simulink model "SM_5_2016a"  (R2016a)
settings: Solver=ode15s  SolverMode=SingleTasking  StartTime=0.001  StopTime=10.0  FixedStep=0.0001  RelTol=1e-6
settings Model: Creator=guaca  LastModifiedBy=Guacamole
settings DebuggingCC: SFUnexpectedBacktrackingDiag=error  SFNoUnconditionalDefaultTransitionDiag=error
settings GRTTargetCC: TargetLangStandard=C99 (ISO)  GeneratePreprocessorConditionals=Use local settings
settings ConfigComp: CovMetricSettings=dwe  CovHtmlReporting=off  CovSaveCumulativeToWorkspaceVar=off  CovSaveSingleToWorkspaceVar=off  CovExternalEMLEnable=on

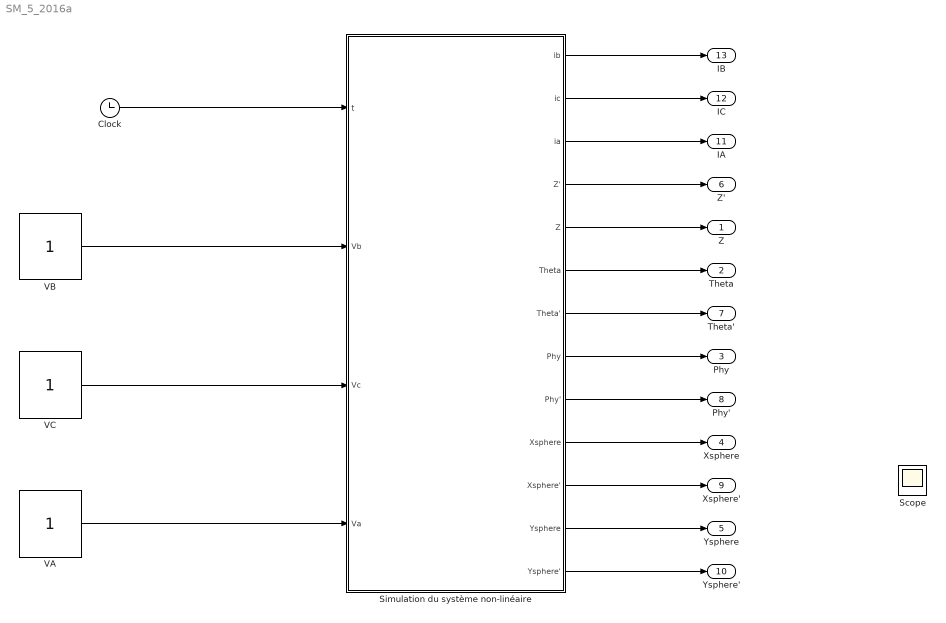
== system SM_5_2016a ==
  Clock : Clock
  Simulation du système non-linéaire : Subsystem
  VA : Constant
  VB : Constant
  VC : Constant
  Z : Outport
  Theta : Outport  Port=2
  Phy : Outport  Port=3
  Xsphere : Outport  Port=4
  Ysphere : Outport  Port=5
  Z' : Outport  Port=6
  Theta' : Outport  Port=7
  Phy' : Outport  Port=8
  Xsphere' : Outport  Port=9
  Ysphere' : Outport  Port=10
  IA : Outport  Port=11
  IC : Outport  Port=12
  IB : Outport  Port=13
  Scope : Scope
  wires:
  Clock/1 -> Simulation du système non-linéaire/1(t)
  VB/1 -> Simulation du système non-linéaire/2(Vb)
  VC/1 -> Simulation du système non-linéaire/3(Vc)
  VA/1 -> Simulation du système non-linéaire/4(Va)
  Simulation du système non-linéaire/1(ib) -> IB/1
  Simulation du système non-linéaire/2(ic) -> IC/1
  Simulation du système non-linéaire/3(ia) -> IA/1
  Simulation du système non-linéaire/4(Z') -> Z'/1
  Simulation du système non-linéaire/5(Z) -> Z/1
  Simulation du système non-linéaire/6(Theta) -> Theta/1
  Simulation du système non-linéaire/7(Theta') -> Theta'/1
  Simulation du système non-linéaire/8(Phy) -> Phy/1
  Simulation du système non-linéaire/9(Phy') -> Phy'/1
  Simulation du système non-linéaire/10(Xsphere) -> Xsphere/1
  Simulation du système non-linéaire/11(Xsphere') -> Xsphere'/1
  Simulation du système non-linéaire/12(Ysphere) -> Ysphere/1
  Simulation du système non-linéaire/13(Ysphere') -> Ysphere'/1

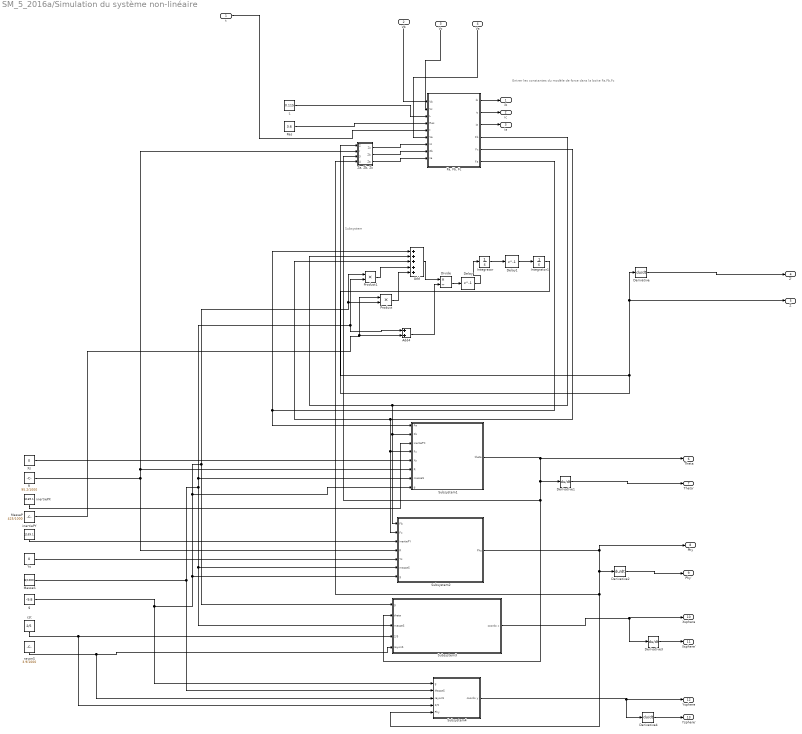
== system SM_5_2016a/Simulation du système non-linéaire ==
  note: Subsystem
  note: Entrer les constantes du modèle de force dans la boite Fa,Fb,Fc
  t : Inport
  Vb : Inport  Port=2
  Vc : Inport  Port=3
  Va : Inport  Port=4
  Add : Sum  Inputs=+++++
  Add4 : Sum
  Delay : Delay  DelayLength=1  InitialCondition=0
  Delay1 : Delay  DelayLength=1  InitialCondition=0
  Derivative{,1..4} (5 alike) : Derivative
  Divide : Product  Inputs=*/
  "Fa, Fb, Fc" : Subsystem
  Integrator : Integrator
  Integrator1 : Integrator
  L : Constant  Value=0.115
  MasseP : Constant  Value=425/1000
  MasseS : Constant  Value=8/1000
  Product : Product
  Product1 : Product
  R : Constant  Value=95.2/1000
  Res : Constant  Value=3.6
  Subsystem1 : Subsystem
  Subsystem2 : Subsystem
  Subsystem3 : Subsystem
  Subsystem4 : Subsystem
  Xs : Constant  Value=0
  Ys : Constant  Value=0
  "Za, Zb, Zc" : Subsystem
  cst : Constant  Value=2/5
  g : Constant  Value=-9.8
  inertiePX : Constant  Value=1169.1
  inertiePY : Constant  Value=1169.1
  rayonS : Constant  Value=3.9/1000
  ib : Outport
  ic : Outport  Port=2
  ia : Outport  Port=3
  Z' : Outport  Port=4
  Z : Outport  Port=5
  Theta : Outport  Port=6
  Theta' : Outport  Port=7
  Phy : Outport  Port=8
  Phy' : Outport  Port=9
  Xsphere : Outport  Port=10
  Xsphere' : Outport  Port=11
  Ysphere : Outport  Port=12
  Ysphere' : Outport  Port=13
  wires:
  rayonS/1 -> Subsystem3/5(rayonS), Subsystem4/3(rayonS)
  R/1 -> Subsystem2/4(R), "Za, Zb, Zc"/2(r), Subsystem1/6(R)
  cst/1 -> Subsystem4/4(2/5), Subsystem3/4(2/5)
  Subsystem1/1(theta) -> Theta/1, "Za, Zb, Zc"/3(Theta), Subsystem3/2(theta), Derivative1/1
  inertiePX/1 -> Subsystem1/3(inertiePX)
  Ys/1 -> Subsystem2/5(Ys)
  Xs/1 -> Subsystem1/5(Xs)
  Subsystem2/1(Phy) -> Phy/1, "Za, Zb, Zc"/4(phy), Subsystem4/5(Phy), Derivative2/1
  Subsystem3/1(coordo x) -> Xsphere/1, Derivative3/1
  Subsystem4/1(coordo y) -> Ysphere/1, Derivative4/1
  inertiePY/1 -> Subsystem2/3(inertiePY)
  Derivative2/1 -> Phy'/1
  t/1 -> "Fa, Fb, Fc"/5(t)
  Va/1 -> "Fa, Fb, Fc"/6(Va)
  Res/1 -> "Fa, Fb, Fc"/4(Res)
  "Fa, Fb, Fc"/2(ic) -> ic/1
  "Fa, Fb, Fc"/3(ia) -> ia/1
  Derivative1/1 -> Theta'/1
  "Fa, Fb, Fc"/1(ib) -> ib/1
  L/1 -> "Fa, Fb, Fc"/3(L)
  Vc/1 -> "Fa, Fb, Fc"/2(Vc)
  Vb/1 -> "Fa, Fb, Fc"/1(Vb)
  Derivative/1 -> Z'/1
  "Za, Zb, Zc"/1(Zc) -> "Fa, Fb, Fc"/7(zc)
  "Za, Zb, Zc"/2(Zb) -> "Fa, Fb, Fc"/8(Zb)
  "Za, Zb, Zc"/3(Za) -> "Fa, Fb, Fc"/9(za)
  Derivative3/1 -> Xsphere'/1
  Integrator1/1 -> Derivative/1, Z/1, "Za, Zb, Zc"/1(Z)
  Derivative4/1 -> Ysphere'/1
  Delay1/1 -> Integrator1/1
  Delay/1 -> Integrator/1
  MasseS/1 -> Subsystem4/2(MasseS), Subsystem3/3(masseS), Subsystem2/6(masseS), Product1/2, Add4/1, Subsystem1/7(masseS)
  g/1 -> Product1/1, Product/2, Subsystem3/1(g), Subsystem1/8(g), Subsystem2/7(g), Subsystem4/1(g)
  "Fa, Fb, Fc"/5(Fc) -> Add/3, Subsystem2/2(Fc), Subsystem1/4(Fc)
  "Fa, Fb, Fc"/4(Fb) -> Add/2, Subsystem2/1(Fb), Subsystem1/2(Fb)
  "Fa, Fb, Fc"/6(Fa) -> Add/1, Subsystem1/1(Fa)
  Add4/1 -> Divide/2
  Add/1 -> Divide/1
  Product1/1 -> Add/4
  Product/1 -> Add/5
  MasseP/1 -> Add4/2, Product/1
  Integrator/1 -> Delay1/1
  Divide/1 -> Delay/1

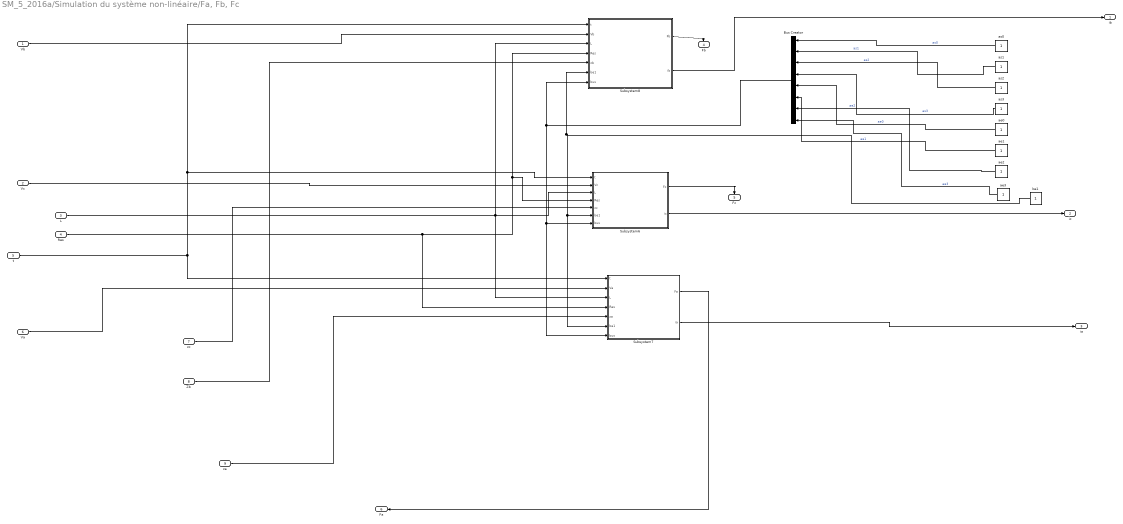
== system SM_5_2016a/Simulation du système non-linéaire/Fa, Fb, Fc ==
  Vb : Inport
  Vc : Inport  Port=2
  L : Inport  Port=3
  Res : Inport  Port=4
  t : Inport  Port=5
  Va : Inport  Port=6
  zc : Inport  Port=7
  Zb : Inport  Port=8
  za : Inport  Port=9
  Bus Creator : BusCreator  Inputs='as0','as1','as2','as3','ae0','ae1','ae2','ae3'
  Subsystem6 : Subsystem
  Subsystem7 : Subsystem
  Subsystem8 : Subsystem
  ae{0..3} (4 alike) : Constant
  as{0..3} (4 alike) : Constant
  be1 : Constant
  ib : Outport
  ic : Outport  Port=2
  ia : Outport  Port=3
  Fb : Outport  Port=4
  Fc : Outport  Port=5
  Fa : Outport  Port=6
  wires:
  ae1/1 -> Bus Creator/6  "ae1"
  ae0/1 -> Bus Creator/5  "ae0"
  as2/1 -> Bus Creator/3  "as2"
  as3/1 -> Bus Creator/4  "as3"
  za/1 -> Subsystem7/5(za)
  Bus Creator/1 -> Subsystem7/7(bus), Subsystem6/7(bus), Subsystem8/7(bus)
  Va/1 -> Subsystem7/2(Va)
  Zb/1 -> Subsystem8/5(zb)
  zc/1 -> Subsystem6/5(zc)
  Subsystem6/1(Fc) -> Fc/1
  be1/1 -> Subsystem7/6(be1), Subsystem6/6(be1), Subsystem8/6(be1)
  Subsystem8/1(Fb) -> Fb/1
  Vb/1 -> Subsystem8/2(Vb)
  Vc/1 -> Subsystem6/2(Vc)
  L/1 -> Subsystem7/3(L), Subsystem6/3(L), Subsystem8/3(L)
  Res/1 -> Subsystem7/4(Res), Subsystem6/4(Res), Subsystem8/4(Res)
  t/1 -> Subsystem8/1(t), Subsystem6/1(t), Subsystem7/1(t)
  as0/1 -> Bus Creator/1  "as0"
  Subsystem7/1(Fa) -> Fa/1
  ae2/1 -> Bus Creator/7  "ae2"
  ae3/1 -> Bus Creator/8  "ae3"
  as1/1 -> Bus Creator/2  "as1"
  Subsystem7/2(ia) -> ia/1
  Subsystem8/2(ib) -> ib/1
  Subsystem6/2(ic) -> ic/1

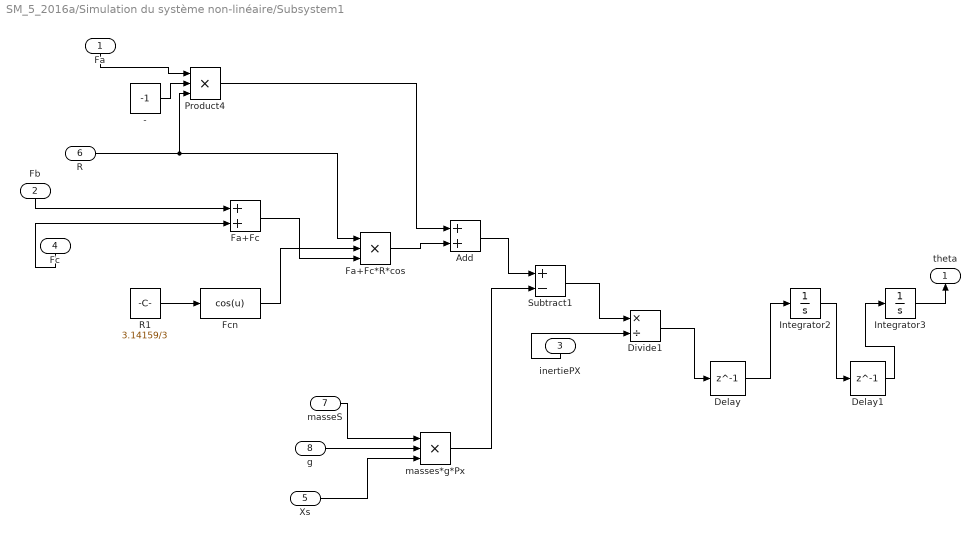
== system SM_5_2016a/Simulation du système non-linéaire/Subsystem1 ==
  Fa : Inport
  Fb : Inport  Port=2
  inertiePX : Inport  Port=3
  Fc : Inport  Port=4
  Xs : Inport  Port=5
  R : Inport  Port=6
  masseS : Inport  Port=7
  g : Inport  Port=8
  - : Constant  Value=-1
  Add : Sum
  Delay : Delay  DelayLength=1  InitialCondition=0
  Delay1 : Delay  DelayLength=1  InitialCondition=0
  Divide1 : Product  Inputs=*/
  Fa+Fc : Sum
  Fa+Fc*R*cos : Product  Inputs=3
  Fcn : Fcn  Expr=cos(u)
  Integrator2 : Integrator
  Integrator3 : Integrator
  Product4 : Product  Inputs=3
  R1 : Constant  Value=3.14159/3
  Subtract1 : Sum  Inputs=+-
  masses*g*Px : Product  Inputs=3
  theta : Outport
  wires:
  Fa+Fc/1 -> Fa+Fc*R*cos/3
  Product4/1 -> Add/1
  -/1 -> Product4/2
  Add/1 -> Subtract1/1
  Subtract1/1 -> Divide1/1
  inertiePX/1 -> Divide1/2
  Divide1/1 -> Delay/1
  Integrator2/1 -> Delay1/1
  Integrator3/1 -> theta/1
  R1/1 -> Fcn/1
  R/1 -> Fa+Fc*R*cos/1, Product4/3
  Fcn/1 -> Fa+Fc*R*cos/2
  Fa+Fc*R*cos/1 -> Add/2
  Xs/1 -> masses*g*Px/3
  masses*g*Px/1 -> Subtract1/2
  masseS/1 -> masses*g*Px/1
  g/1 -> masses*g*Px/2
  Fc/1 -> Fa+Fc/2
  Fb/1 -> Fa+Fc/1
  Fa/1 -> Product4/1
  Delay/1 -> Integrator2/1
  Delay1/1 -> Integrator3/1

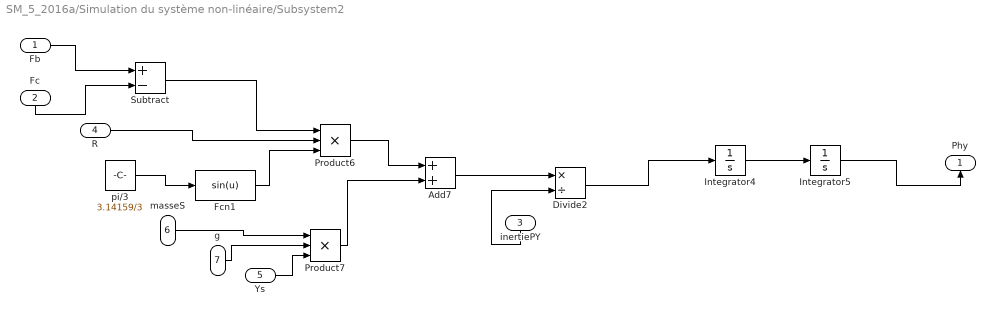
== system SM_5_2016a/Simulation du système non-linéaire/Subsystem2 ==
  Fb : Inport
  Fc : Inport  Port=2
  inertiePY : Inport  Port=3
  R : Inport  Port=4
  Ys : Inport  Port=5
  masseS : Inport  Port=6
  g : Inport  Port=7
  Add7 : Sum
  Divide2 : Product  Inputs=*/
  Fcn1 : Fcn  Expr=sin(u)
  Integrator4 : Integrator
  Integrator5 : Integrator
  Product6 : Product  Inputs=3
  Product7 : Product  Inputs=3
  Subtract : Sum  Inputs=+-
  pi/3 : Constant  Value=3.14159/3
  Phy : Outport
  wires:
  Fcn1/1 -> Product6/3
  pi/3/1 -> Fcn1/1
  Subtract/1 -> Product6/1
  Product6/1 -> Add7/1
  Product7/1 -> Add7/2
  Add7/1 -> Divide2/1
  inertiePY/1 -> Divide2/2
  Divide2/1 -> Integrator4/1
  Integrator4/1 -> Integrator5/1
  Integrator5/1 -> Phy/1
  masseS/1 -> Product7/1
  Fc/1 -> Subtract/2
  Ys/1 -> Product7/3
  R/1 -> Product6/2
  g/1 -> Product7/2
  Fb/1 -> Subtract/1

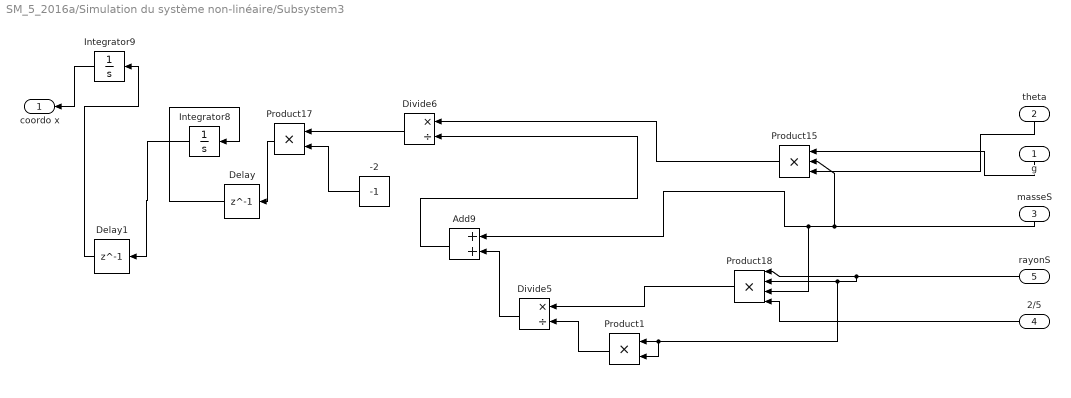
== system SM_5_2016a/Simulation du système non-linéaire/Subsystem3 ==
  g : Inport
  theta : Inport  Port=2
  masseS : Inport  Port=3
  2/5 : Inport  Port=4
  rayonS : Inport  Port=5
  -2 : Constant  Value=-1
  Add9 : Sum
  Delay : Delay  DelayLength=1  InitialCondition=0
  Delay1 : Delay  DelayLength=1  InitialCondition=0
  Divide5 : Product  Inputs=*/
  Divide6 : Product  Inputs=*/
  Integrator8 : Integrator
  Integrator9 : Integrator
  Product1 : Product
  Product15 : Product  Inputs=3
  Product17 : Product
  Product18 : Product  Inputs=4
  coordo x : Outport
  wires:
  Product18/1 -> Divide5/1
  Divide5/1 -> Add9/2
  Product15/1 -> Divide6/1
  Add9/1 -> Divide6/2
  Integrator8/1 -> Delay1/1
  Integrator9/1 -> coordo x/1
  Divide6/1 -> Product17/1
  -2/1 -> Product17/2
  masseS/1 -> Product15/2, Add9/1, Product18/3
  rayonS/1 -> Product1/2, Product1/1, Product18/2, Product18/1
  2/5/1 -> Product18/4
  g/1 -> Product15/1
  theta/1 -> Product15/3
  Product17/1 -> Delay/1
  Delay/1 -> Integrator8/1
  Delay1/1 -> Integrator9/1
  Product1/1 -> Divide5/2

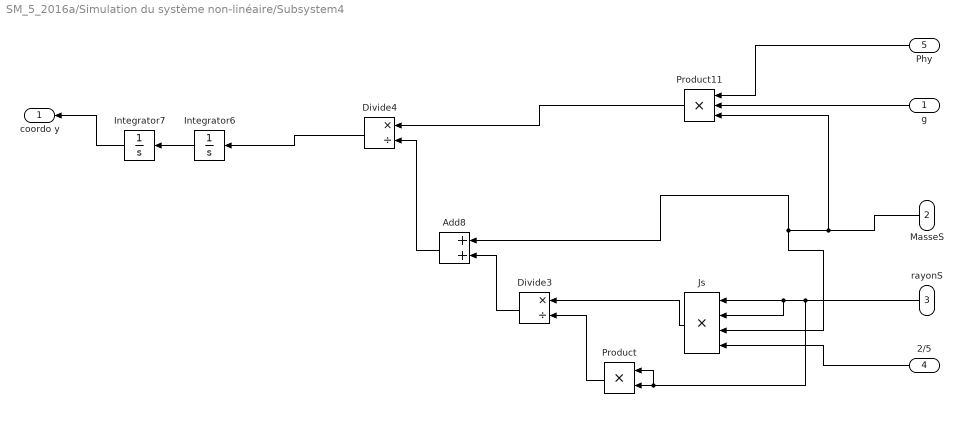
== system SM_5_2016a/Simulation du système non-linéaire/Subsystem4 ==
  g : Inport
  MasseS : Inport  Port=2
  rayonS : Inport  Port=3
  2/5 : Inport  Port=4
  Phy : Inport  Port=5
  Add8 : Sum
  Divide3 : Product  Inputs=*/
  Divide4 : Product  Inputs=*/
  Integrator6 : Integrator
  Integrator7 : Integrator
  Js : Product  Inputs=4
  Product : Product
  Product11 : Product  Inputs=3
  coordo y : Outport
  wires:
  Js/1 -> Divide3/1
  Divide3/1 -> Add8/2
  Product11/1 -> Divide4/1
  Add8/1 -> Divide4/2
  Integrator6/1 -> Integrator7/1
  Integrator7/1 -> coordo y/1
  Divide4/1 -> Integrator6/1
  g/1 -> Product11/2
  rayonS/1 -> Product/1, Product/2, Js/2, Js/1
  2/5/1 -> Js/4
  Phy/1 -> Product11/1
  MasseS/1 -> Product11/3, Js/3, Add8/1
  Product/1 -> Divide3/2

== system SM_5_2016a/Simulation du système non-linéaire/Za, Zb, Zc ==
  Z : Inport
  r : Inport  Port=2
  Theta : Inport  Port=3
  phy : Inport  Port=4
  Subsystem10 : Subsystem
  Subsystem5 : Subsystem
  Subsystem9 : Subsystem
  Zc : Outport
  Zb : Outport  Port=2
  Za : Outport  Port=3
  wires:
  Subsystem5/1(Za) -> Za/1
  Subsystem10/1(Zc) -> Zc/1
  Subsystem9/1(Zb) -> Zb/1
  r/1 -> Subsystem10/3(r), Subsystem9/3(r), Subsystem5/3(R)
  phy/1 -> Subsystem10/4(phy), Subsystem9/4(phy)
  Z/1 -> Subsystem10/1(Z), Subsystem9/1(Z), Subsystem5/1(Z)
  Theta/1 -> Subsystem10/2(theta), Subsystem9/2(theta), Subsystem5/2(theta)

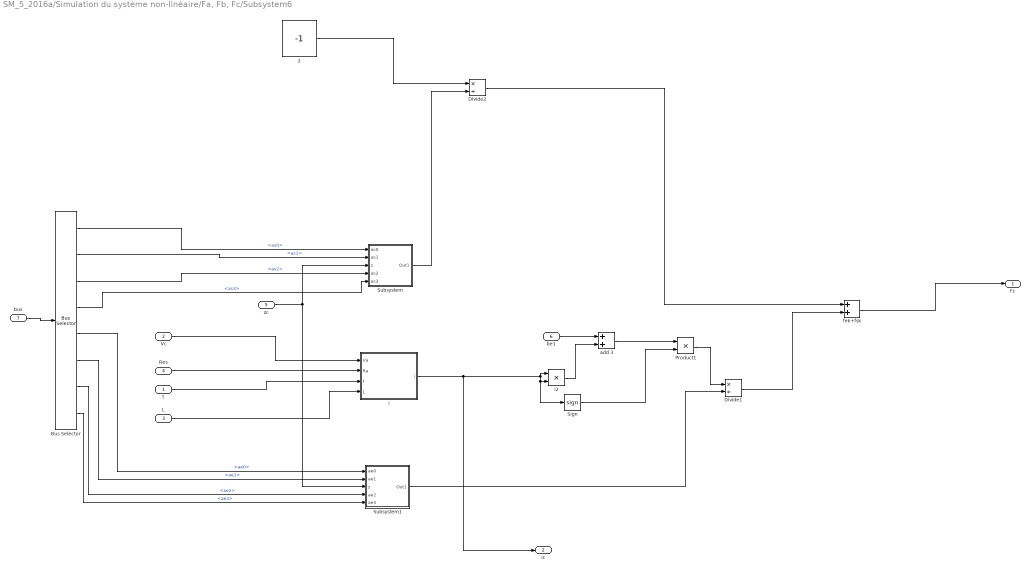
== system SM_5_2016a/Simulation du système non-linéaire/Fa, Fb, Fc/Subsystem6 ==
  t : Inport
  Vc : Inport  Port=2
  L : Inport  Port=3
  Res : Inport  Port=4
  zc : Inport  Port=5
  be1 : Inport  Port=6
  bus : Inport  Port=7
  2 : Constant  Value=-1
  Bus Selector : BusSelector  OutputSignals=as0,as1,as2,as3,ae0,ae1,ae2,ae3
  Divide1 : Product  Inputs=*/
  Divide2 : Product  Inputs=*/
  Product1 : Product
  Sign : Signum
  Subsystem : Subsystem
  Subsystem1 : Subsystem
  add 3 : Sum
  fek+fsk : Sum
  i : Subsystem
  i2 : Product
  Fc : Outport
  ic : Outport  Port=2
  wires:
  fek+fsk/1 -> Fc/1
  2/1 -> Divide2/1
  Divide2/1 -> fek+fsk/1
  i2/1 -> add 3/2
  i/1(i) -> ic/1, Sign/1, i2/2, i2/1
  Vc/1 -> i/1(Va)
  Res/1 -> i/2(Ra)
  t/1 -> i/3(t)
  L/1 -> i/4(L)
  be1/1 -> add 3/1
  add 3/1 -> Product1/1
  Sign/1 -> Product1/2
  Bus Selector/1 -> Subsystem/1(as0)  "<as0>"
  Bus Selector/2 -> Subsystem/2(as1)  "<as1>"
  zc/1 -> Subsystem/3(z), Subsystem1/3(z)
  Bus Selector/3 -> Subsystem/4(as2)  "<as2>"
  Bus Selector/4 -> Subsystem/5(as3)  "<as3>"
  Subsystem/1(Out1) -> Divide2/2
  Bus Selector/5 -> Subsystem1/1(ae0)  "<ae0>"
  Bus Selector/6 -> Subsystem1/2(ae1)  "<ae1>"
  Bus Selector/7 -> Subsystem1/4(ae2)  "<ae2>"
  Bus Selector/8 -> Subsystem1/5(ae3)  "<ae3>"
  Subsystem1/1(Out1) -> Divide1/2
  Product1/1 -> Divide1/1
  Divide1/1 -> fek+fsk/2
  bus/1 -> Bus Selector/1

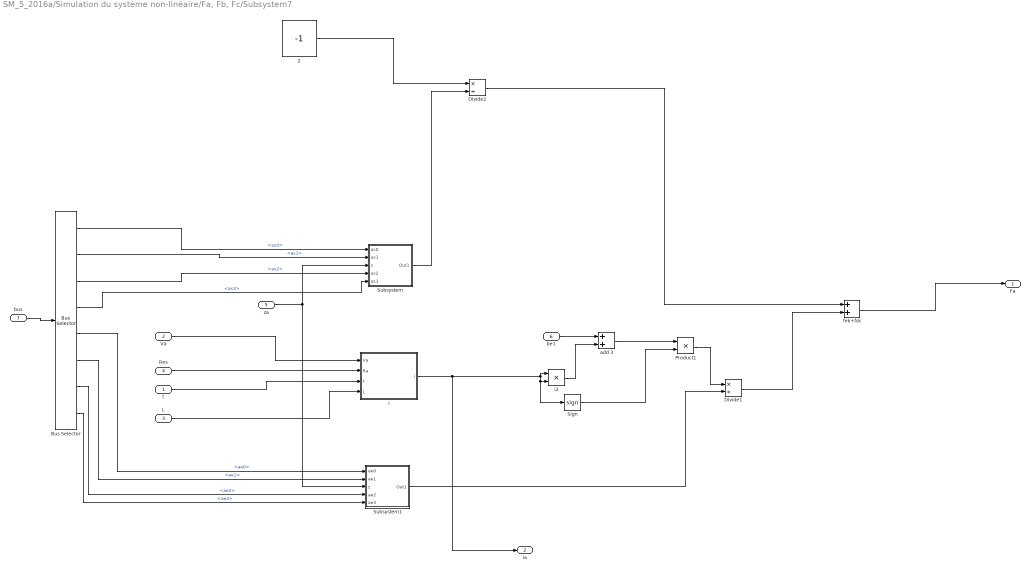
== system SM_5_2016a/Simulation du système non-linéaire/Fa, Fb, Fc/Subsystem7 ==
  t : Inport
  Va : Inport  Port=2
  L : Inport  Port=3
  Res : Inport  Port=4
  za : Inport  Port=5
  be1 : Inport  Port=6
  bus : Inport  Port=7
  2 : Constant  Value=-1
  Bus Selector : BusSelector  OutputSignals=as0,as1,as2,as3,ae0,ae1,ae2,ae3
  Divide1 : Product  Inputs=*/
  Divide2 : Product  Inputs=*/
  Product1 : Product
  Sign : Signum
  Subsystem : Subsystem
  Subsystem1 : Subsystem
  add 3 : Sum
  fek+fsk : Sum
  i : Subsystem
  i2 : Product
  Fa : Outport
  ia : Outport  Port=2
  wires:
  fek+fsk/1 -> Fa/1
  2/1 -> Divide2/1
  Divide2/1 -> fek+fsk/1
  i2/1 -> add 3/2
  i/1(i) -> ia/1, Sign/1, i2/2, i2/1
  Va/1 -> i/1(Va)
  Res/1 -> i/2(Ra)
  t/1 -> i/3(t)
  L/1 -> i/4(L)
  be1/1 -> add 3/1
  add 3/1 -> Product1/1
  Sign/1 -> Product1/2
  Bus Selector/1 -> Subsystem/1(as0)  "<as0>"
  Bus Selector/2 -> Subsystem/2(as1)  "<as1>"
  za/1 -> Subsystem/3(z), Subsystem1/3(z)
  Bus Selector/3 -> Subsystem/4(as2)  "<as2>"
  Bus Selector/4 -> Subsystem/5(as3)  "<as3>"
  Subsystem/1(Out1) -> Divide2/2
  Bus Selector/5 -> Subsystem1/1(ae0)  "<ae0>"
  Bus Selector/6 -> Subsystem1/2(ae1)  "<ae1>"
  Bus Selector/7 -> Subsystem1/4(ae2)  "<ae2>"
  Bus Selector/8 -> Subsystem1/5(ae3)  "<ae3>"
  Subsystem1/1(Out1) -> Divide1/2
  Product1/1 -> Divide1/1
  Divide1/1 -> fek+fsk/2
  bus/1 -> Bus Selector/1

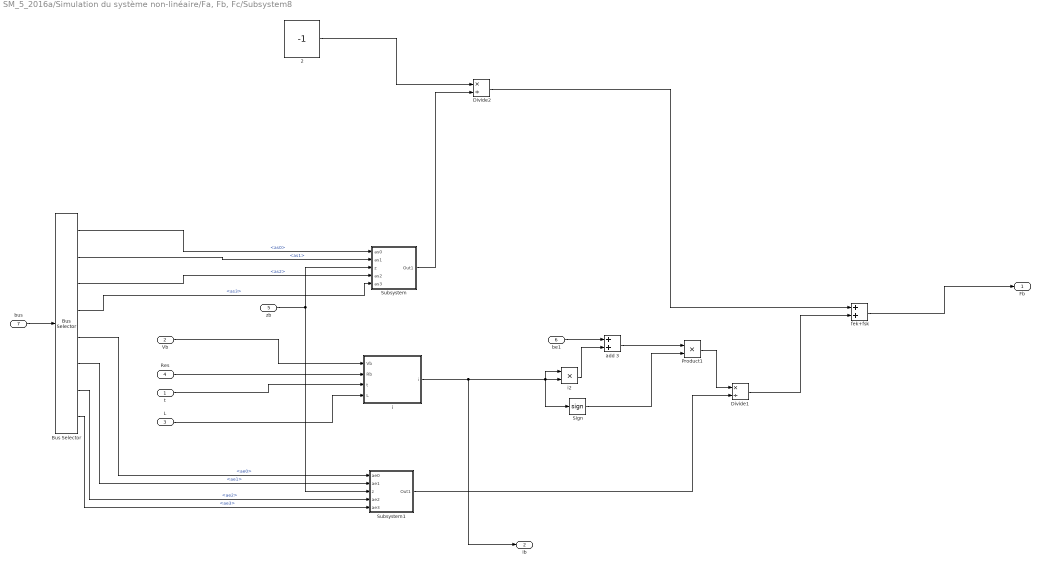
== system SM_5_2016a/Simulation du système non-linéaire/Fa, Fb, Fc/Subsystem8 ==
  t : Inport
  Vb : Inport  Port=2
  L : Inport  Port=3
  Res : Inport  Port=4
  zb : Inport  Port=5
  be1 : Inport  Port=6
  bus : Inport  Port=7
  2 : Constant  Value=-1
  Bus Selector : BusSelector  OutputSignals=as0,as1,as2,as3,ae0,ae1,ae2,ae3
  Divide1 : Product  Inputs=*/
  Divide2 : Product  Inputs=*/
  Product1 : Product
  Sign : Signum
  Subsystem : Subsystem
  Subsystem1 : Subsystem
  add 3 : Sum
  fek+fsk : Sum
  i : Subsystem
  i2 : Product
  Fb : Outport
  ib : Outport  Port=2
  wires:
  fek+fsk/1 -> Fb/1
  2/1 -> Divide2/1
  Divide2/1 -> fek+fsk/1
  i2/1 -> add 3/2
  i/1(i) -> ib/1, Sign/1, i2/2, i2/1
  Vb/1 -> i/1(Vb)
  Res/1 -> i/2(Rb)
  t/1 -> i/3(t)
  L/1 -> i/4(L)
  be1/1 -> add 3/1
  add 3/1 -> Product1/1
  Sign/1 -> Product1/2
  Bus Selector/1 -> Subsystem/1(as0)  "<as0>"
  Bus Selector/2 -> Subsystem/2(as1)  "<as1>"
  zb/1 -> Subsystem/3(z), Subsystem1/3(z)
  Bus Selector/3 -> Subsystem/4(as2)  "<as2>"
  Bus Selector/4 -> Subsystem/5(as3)  "<as3>"
  Subsystem/1(Out1) -> Divide2/2
  Bus Selector/5 -> Subsystem1/1(ae0)  "<ae0>"
  Bus Selector/6 -> Subsystem1/2(ae1)  "<ae1>"
  Bus Selector/7 -> Subsystem1/4(ae2)  "<ae2>"
  Bus Selector/8 -> Subsystem1/5(ae3)  "<ae3>"
  Subsystem1/1(Out1) -> Divide1/2
  Product1/1 -> Divide1/1
  Divide1/1 -> fek+fsk/2
  bus/1 -> Bus Selector/1

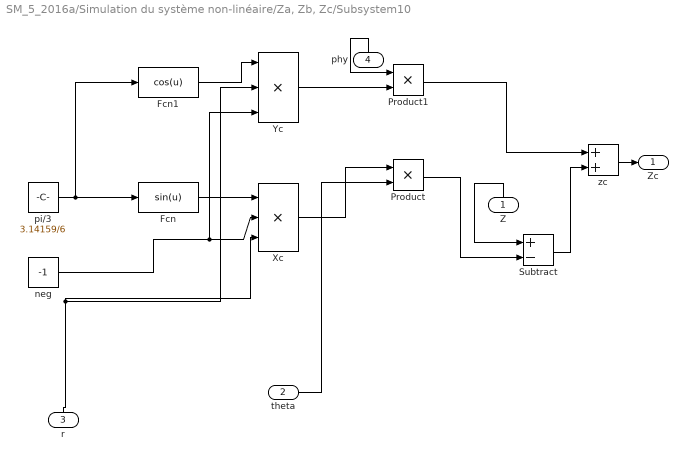
== system SM_5_2016a/Simulation du système non-linéaire/Za, Zb, Zc/Subsystem10 ==
  Z : Inport
  theta : Inport  Port=2
  r : Inport  Port=3
  phy : Inport  Port=4
  Fcn : Fcn  Expr=sin(u)
  Fcn1 : Fcn  Expr=cos(u)
  Product : Product
  Product1 : Product
  Subtract : Sum  Inputs=+-
  Xc : Product  Inputs=3
  Yc : Product  Inputs=3
  neg : Constant  Value=-1
  pi/3 : Constant  Value=3.14159/6
  zc : Sum
  Zc : Outport
  wires:
  Fcn1/1 -> Yc/1
  Xc/1 -> Product/1
  neg/1 -> Yc/3, Xc/2
  phy/1 -> Product1/1
  r/1 -> Yc/2, Xc/3
  zc/1 -> Zc/1
  Product1/1 -> zc/1
  Z/1 -> Subtract/1
  theta/1 -> Product/2
  Fcn/1 -> Xc/1
  pi/3/1 -> Fcn1/1, Fcn/1
  Product/1 -> Subtract/2
  Subtract/1 -> zc/2
  Yc/1 -> Product1/2

== system SM_5_2016a/Simulation du système non-linéaire/Za, Zb, Zc/Subsystem5 ==
  Z : Inport
  theta : Inport  Port=2
  R : Inport  Port=3
  Product : Product
  Subtract : Sum  Inputs=+-
  Za : Outport
  wires:
  Product/1 -> Subtract/2
  Subtract/1 -> Za/1
  Z/1 -> Subtract/1
  R/1 -> Product/1
  theta/1 -> Product/2

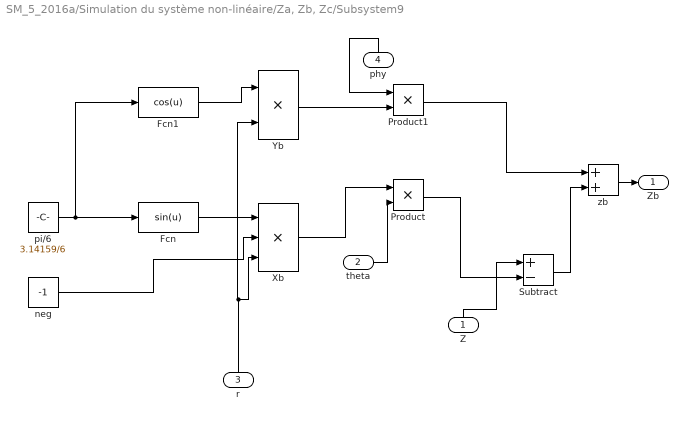
== system SM_5_2016a/Simulation du système non-linéaire/Za, Zb, Zc/Subsystem9 ==
  Z : Inport
  theta : Inport  Port=2
  r : Inport  Port=3
  phy : Inport  Port=4
  Fcn : Fcn  Expr=sin(u)
  Fcn1 : Fcn  Expr=cos(u)
  Product : Product
  Product1 : Product
  Subtract : Sum  Inputs=+-
  Xb : Product  Inputs=3
  Yb : Product
  neg : Constant  Value=-1
  pi/6 : Constant  Value=3.14159/6
  zb : Sum
  Zb : Outport
  wires:
  Fcn1/1 -> Yb/1
  Xb/1 -> Product/1
  neg/1 -> Xb/2
  phy/1 -> Product1/1
  r/1 -> Yb/2, Xb/3
  zb/1 -> Zb/1
  Product1/1 -> zb/1
  Z/1 -> Subtract/1
  theta/1 -> Product/2
  Fcn/1 -> Xb/1
  pi/6/1 -> Fcn1/1, Fcn/1
  Product/1 -> Subtract/2
  Subtract/1 -> zb/2
  Yb/1 -> Product1/2

== system SM_5_2016a/Simulation du système non-linéaire/Fa, Fb, Fc/Subsystem6/Subsystem ==
  as0 : Inport
  as1 : Inport  Port=2
  z : Inport  Port=3
  as2 : Inport  Port=4
  as3 : Inport  Port=5
  Add : Sum  Inputs=++++
  Product4 : Product
  Product5 : Product  Inputs=3
  Product6 : Product  Inputs=4
  Out1 : Outport
  wires:
  as0/1 -> Add/1
  Product5/1 -> Add/3
  Product4/1 -> Add/2
  Product6/1 -> Add/4
  z/1 -> Product5/3, Product6/1, Product6/4, Product6/3, Product5/1, Product4/1
  as1/1 -> Product4/2
  as2/1 -> Product5/2
  as3/1 -> Product6/2
  Add/1 -> Out1/1

== system SM_5_2016a/Simulation du système non-linéaire/Fa, Fb, Fc/Subsystem6/Subsystem1 ==
  ae0 : Inport
  ae1 : Inport  Port=2
  z : Inport  Port=3
  ae2 : Inport  Port=4
  ae3 : Inport  Port=5
  Add : Sum  Inputs=++++
  Product4 : Product
  Product5 : Product  Inputs=3
  Product6 : Product  Inputs=4
  Out1 : Outport
  wires:
  ae0/1 -> Add/1
  Product5/1 -> Add/3
  Product4/1 -> Add/2
  Product6/1 -> Add/4
  z/1 -> Product5/3, Product6/1, Product6/4, Product6/3, Product5/1, Product4/1
  ae1/1 -> Product4/2
  ae2/1 -> Product5/2
  ae3/1 -> Product6/2
  Add/1 -> Out1/1

== system SM_5_2016a/Simulation du système non-linéaire/Fa, Fb, Fc/Subsystem6/i ==
  Va : Inport
  Ra : Inport  Port=2
  t : Inport  Port=3
  L : Inport  Port=4
  1 : Constant
  3 : Constant  Value=-1
  Divide1 : Product  Inputs=*/
  Divide8 : Product  Inputs=*/
  Math Function : Math  SaturateOnIntegerOverflow=on
  Product1 : Product
  Product20 : Product
  Product3 : Product
  Subtract2 : Sum  Inputs=+-
  i : Outport
  wires:
  1/1 -> Subtract2/1
  Math Function/1 -> Subtract2/2
  Divide8/1 -> Math Function/1
  Va/1 -> Divide1/1
  Ra/1 -> Product20/1, Divide1/2
  t/1 -> Product20/2
  Product20/1 -> Divide8/1
  L/1 -> Product1/1
  3/1 -> Product1/2
  Product1/1 -> Divide8/2
  Divide1/1 -> Product3/1
  Subtract2/1 -> Product3/2
  Product3/1 -> i/1  "i"

== system SM_5_2016a/Simulation du système non-linéaire/Fa, Fb, Fc/Subsystem7/Subsystem ==
  as0 : Inport
  as1 : Inport  Port=2
  z : Inport  Port=3
  as2 : Inport  Port=4
  as3 : Inport  Port=5
  Add : Sum  Inputs=++++
  Product4 : Product
  Product5 : Product  Inputs=3
  Product6 : Product  Inputs=4
  Out1 : Outport
  wires:
  as0/1 -> Add/1
  Product5/1 -> Add/3
  Product4/1 -> Add/2
  Product6/1 -> Add/4
  z/1 -> Product5/3, Product6/1, Product6/4, Product6/3, Product5/1, Product4/1
  as1/1 -> Product4/2
  as2/1 -> Product5/2
  as3/1 -> Product6/2
  Add/1 -> Out1/1

== system SM_5_2016a/Simulation du système non-linéaire/Fa, Fb, Fc/Subsystem7/Subsystem1 ==
  ae0 : Inport
  ae1 : Inport  Port=2
  z : Inport  Port=3
  ae2 : Inport  Port=4
  ae3 : Inport  Port=5
  Add : Sum  Inputs=++++
  Product4 : Product
  Product5 : Product  Inputs=3
  Product6 : Product  Inputs=4
  Out1 : Outport
  wires:
  ae0/1 -> Add/1
  Product5/1 -> Add/3
  Product4/1 -> Add/2
  Product6/1 -> Add/4
  z/1 -> Product5/3, Product6/1, Product6/4, Product6/3, Product5/1, Product4/1
  ae1/1 -> Product4/2
  ae2/1 -> Product5/2
  ae3/1 -> Product6/2
  Add/1 -> Out1/1

== system SM_5_2016a/Simulation du système non-linéaire/Fa, Fb, Fc/Subsystem7/i ==
  Va : Inport
  Ra : Inport  Port=2
  t : Inport  Port=3
  L : Inport  Port=4
  1 : Constant
  3 : Constant  Value=-1
  Divide1 : Product  Inputs=*/
  Divide8 : Product  Inputs=*/
  Math Function : Math  SaturateOnIntegerOverflow=on
  Product1 : Product
  Product20 : Product
  Product3 : Product
  Subtract2 : Sum  Inputs=+-
  i : Outport
  wires:
  1/1 -> Subtract2/1
  Math Function/1 -> Subtract2/2
  Divide8/1 -> Math Function/1
  Va/1 -> Divide1/1
  Ra/1 -> Product20/1, Divide1/2
  t/1 -> Product20/2
  Product20/1 -> Divide8/1
  L/1 -> Product1/1
  3/1 -> Product1/2
  Product1/1 -> Divide8/2
  Divide1/1 -> Product3/1
  Subtract2/1 -> Product3/2
  Product3/1 -> i/1  "i"

== system SM_5_2016a/Simulation du système non-linéaire/Fa, Fb, Fc/Subsystem8/Subsystem ==
  as0 : Inport
  as1 : Inport  Port=2
  z : Inport  Port=3
  as2 : Inport  Port=4
  as3 : Inport  Port=5
  Add : Sum  Inputs=++++
  Product4 : Product
  Product5 : Product  Inputs=3
  Product6 : Product  Inputs=4
  Out1 : Outport
  wires:
  as0/1 -> Add/1
  Product5/1 -> Add/3
  Product4/1 -> Add/2
  Product6/1 -> Add/4
  z/1 -> Product5/3, Product6/1, Product6/4, Product6/3, Product5/1, Product4/1
  as1/1 -> Product4/2
  as2/1 -> Product5/2
  as3/1 -> Product6/2
  Add/1 -> Out1/1

== system SM_5_2016a/Simulation du système non-linéaire/Fa, Fb, Fc/Subsystem8/Subsystem1 ==
  ae0 : Inport
  ae1 : Inport  Port=2
  z : Inport  Port=3
  ae2 : Inport  Port=4
  ae3 : Inport  Port=5
  Add : Sum  Inputs=++++
  Product4 : Product
  Product5 : Product  Inputs=3
  Product6 : Product  Inputs=4
  Out1 : Outport
  wires:
  ae0/1 -> Add/1
  Product5/1 -> Add/3
  Product4/1 -> Add/2
  Product6/1 -> Add/4
  z/1 -> Product5/3, Product6/1, Product6/4, Product6/3, Product5/1, Product4/1
  ae1/1 -> Product4/2
  ae2/1 -> Product5/2
  ae3/1 -> Product6/2
  Add/1 -> Out1/1

== system SM_5_2016a/Simulation du système non-linéaire/Fa, Fb, Fc/Subsystem8/i ==
  Vb : Inport
  Rb : Inport  Port=2
  t : Inport  Port=3
  L : Inport  Port=4
  1 : Constant
  3 : Constant  Value=-1
  Divide1 : Product  Inputs=*/
  Divide8 : Product  Inputs=*/
  Math Function : Math  SaturateOnIntegerOverflow=on
  Product1 : Product
  Product20 : Product
  Product3 : Product
  Subtract2 : Sum  Inputs=+-
  i : Outport
  wires:
  1/1 -> Subtract2/1
  Math Function/1 -> Subtract2/2
  Divide8/1 -> Math Function/1
  Vb/1 -> Divide1/1
  Rb/1 -> Product20/1, Divide1/2
  t/1 -> Product20/2
  Product20/1 -> Divide8/1
  L/1 -> Product1/1
  3/1 -> Product1/2
  Product1/1 -> Divide8/2
  Divide1/1 -> Product3/1
  Subtract2/1 -> Product3/2
  Product3/1 -> i/1  "i"
